simulink model "Basic_DSB_SC"  (R2017a)
settings: Solver=VariableStepAuto  StartTime=0.0  StopTime=inf  RelTol=1e-3
libraries: commanapbnd3 x1
settings Model: Creator=Mike  LastModifiedBy=Mike
settings DataIOCC: LimitDataPoints=on  SaveOutput=off  SaveTime=off
settings OptimizationCC: BlockReduction=off  BooleanDataType=off  LifeSpan=inf
settings DebuggingCC: SaveWithParameterizedLinksMsg=none  UnderspecifiedInitializationDetection=Classic  MergeDetectMultiDrivingBlocksExec=none  SignalResolutionControl=TryResolveAllWithWarning  AllowSymbolicDim=off  SFUnexpectedBacktrackingDiag=warning  SFNoUnconditionalDefaultTransitionDiag=warning  SFExecutionAtInitializationDiag=none
settings HardwareCC: TargetUnknown=on
settings GRTTargetCC: TargetLangStandard=C89/C90 (ANSI)  GeneratePreprocessorConditionals=Disable all

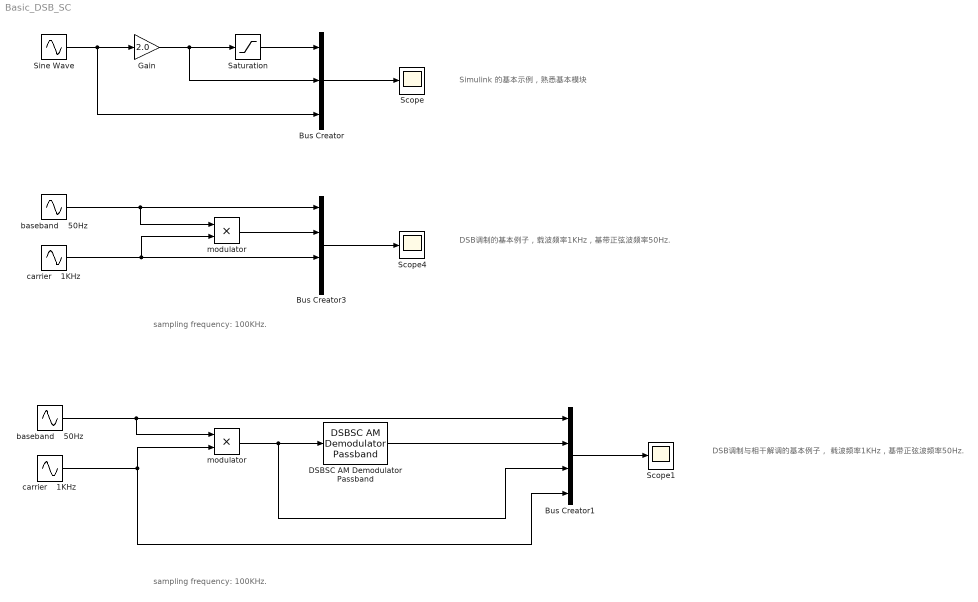
== system Basic_DSB_SC ==
  note: Simulink 的基本示例，熟悉基本模块
  note: DSB调制的基本例子，载波频率1KHz，基带正弦波频率50Hz.
  note: sampling frequency: 100KHz.
  note: sampling frequency: 100KHz.
  note: DSB调制与相干解调的基本例子，
      |
      | 载波频率1KHz，基带正弦波频率50Hz.
  Bus Creator : BusCreator  Inputs=3
  Bus Creator1 : BusCreator  Inputs=4
  Bus Creator3 : BusCreator  Inputs=4
  DSBSC AM Demodulator Passband : commanapbnd3/DSBSC AM Demodulator Passband  Fc=1000  Ph=0  method=Butterworth  n=4  cf=100  Rp=0.1  Rs=50
      settings: SourceProductName=Communications System Toolbox  SourceProductBaseCode=CM
  Gain : Gain  Gain=2.0
  Saturation : Saturate
  Scope : Scope
  Scope1 : Scope
  Scope4 : Scope
  Sine Wave : Sin  SampleTime=0
  baseband    50Hz : Sin  SineType=Sample based  Samples=2e3  SampleTime=1e-5  Offset=5e2
  "baseband    50Hz  " : Sin  SineType=Sample based  Samples=2e3  SampleTime=1e-5  Offset=5e2
  carrier    1KHz : Sin  SineType=Sample based  Samples=1e2  SampleTime=1e-5  Offset=25
  "carrier    1KHz  " : Sin  SineType=Sample based  Samples=1e2  SampleTime=1e-5  Offset=25
  modulator : Product  Inputs=**
  "modulator  " : Product  Inputs=**
  wires:
  Gain/1 -> Bus Creator/2, Saturation/1
  Sine Wave/1 -> Bus Creator/3, Gain/1
  Bus Creator/1 -> Scope/1
  Saturation/1 -> Bus Creator/1
  carrier    1KHz/1 -> Bus Creator3/3, modulator/2
  Bus Creator3/1 -> Scope4/1
  baseband    50Hz/1 -> Bus Creator3/1, modulator/1
  modulator/1 -> Bus Creator3/2
  "baseband    50Hz  "/1 -> Bus Creator1/1, "modulator  "/1
  "carrier    1KHz  "/1 -> Bus Creator1/4, "modulator  "/2
  "modulator  "/1 -> Bus Creator1/3, DSBSC AM Demodulator Passband/1
  DSBSC AM Demodulator Passband/1 -> Bus Creator1/2
  Bus Creator1/1 -> Scope1/1
